simulink model "simulation_base"  (R2013a)
settings: Solver=ode4  StartTime=0.0  StopTime=10  FixedStep=Ts  RelTol=1e-3
values from neighbouring files (symbols this model uses):
  Cdc = 5e-3    (= 0.005)    [rpg_simulation_base.m]
  Crpcu_each = 1/(2*pi*fs*Zrpcu_each)    [rpg_simulation_base.m]
  ESR = 1e-3    (= 0.001)    [rpg_simulation_base.m]
  fs = 50    [rpg_loss_calculation.m]    (also in rpg_simulation_base.m)
  Lload = Xload/wout    [rpg_simulation_base.m]
  Ls = 1e-3    (= 0.001)    [rpg_simulation_base.m]
  Ppv = 40e3    (= 40000)    [rpg_simulation_base.m]
  Qpv = 30e3    (= 30000)    [rpg_simulation_base.m]
  Rload = Zload*pf    [rpg_simulation_base.m]
  RLs = 10e-3    (= 0.01)    [rpg_simulation_base.m]
  Rseries = 5    [rpg_simulation_base.m]
  Ts = 1e-5    (= 1e-05)    [rpg_simulation_base.m]
  V1 = Vdc*(Rseries+Rrefl)/Rrefl    (= 1083.33333333)    [rpg_simulation_base.m]
  Vdc = 750    [calculate_loss.m]    (also in rpg_loss_calculation.m; rpg_simulation_base.m)
  Vline = 400    [calculate_loss.m]    (also in rpg_loss_calculation.m; rpg_simulation_base.m = 34500)
  Vphase = 400/sqrt(3)    [rpg_simulation_base.m]
  Xs = 2*pi*fs*Ls    (= 0.314159265359)    [rpg_simulation_base.m]
undefined symbols (not defined in the file or in its folder): rpcu_s1, rpcu_s2, rpcu_s3, rpcu_s4
libraries: powerlib x74, powerlib_meascontrol x13, simulink x1
settings Model: Creator=hp  LastModifiedBy=ugurm

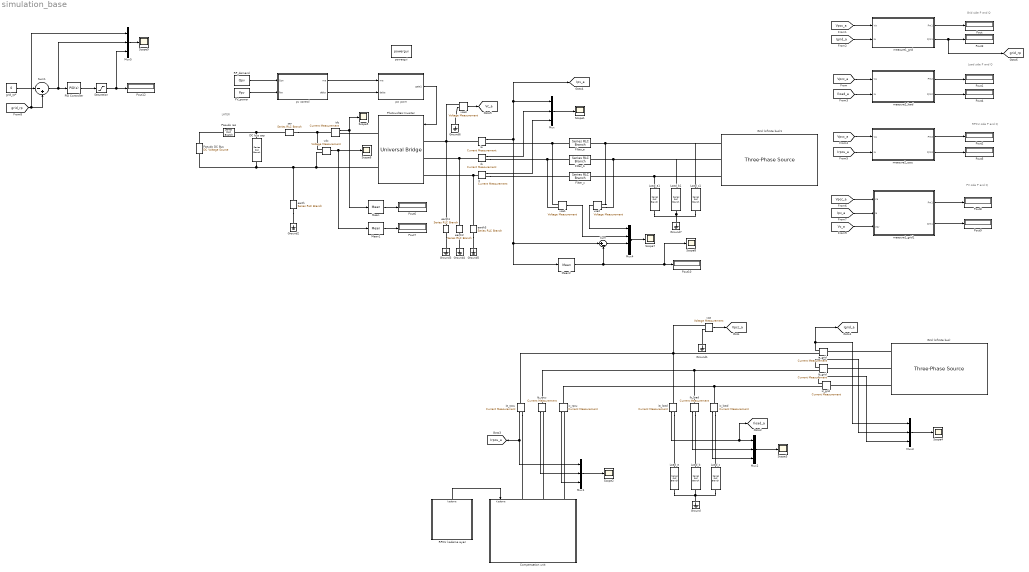
== system simulation_base ==
  note: LATER
  note: Grid side P and Q
  note: Load side P and Q
  note: RPCU side P and Q
  note: PV side P and Q
  Compensation unit : Subsystem
  DC bus cap : powerlib/Elements/Series RLC Branch  LConnTagsString=__new0  RConnTagsString=__new0  BranchType=RC  Resistance=ESR  Inductance=1e-3  SetiL0=off  InitialCurrent=0  Capacitance=Cdc  Setx0=on  InitialVoltage=600  Measurements=None
  Filter_a : powerlib/Elements/Series RLC Branch  LConnTagsString=__new0  RConnTagsString=__new0  BranchType=RL  Resistance=RLs  Inductance=Ls  SetiL0=off  InitialCurrent=0  Capacitance=1e-6  Setx0=off  InitialVoltage=0  Measurements=None
  Filter_b : powerlib/Elements/Series RLC Branch  LConnTagsString=__new0  RConnTagsString=__new0  BranchType=RL  Resistance=RLs  Inductance=Ls  SetiL0=off  InitialCurrent=0  Capacitance=1e-6  Setx0=off  InitialVoltage=0  Measurements=None
  Filter_c : powerlib/Elements/Series RLC Branch  LConnTagsString=__new0  RConnTagsString=__new0  BranchType=RL  Resistance=RLs  Inductance=Ls  SetiL0=off  InitialCurrent=0  Capacitance=1e-6  Setx0=off  InitialVoltage=0  Measurements=None
  Grid (infinite bus) : powerlib/Electrical Sources/Three-Phase Source  Voltage=Vline  PhaseAngle=0  Frequency=fs  InternalConnection=Yg  SpecifyImpedance=off  Resistance=0  Inductance=0  ShortCircuitLevel=100e6  BaseVoltage=Vline  XRratio=7  BusType=swing  Pref=0  Qref=0  Qmin=-inf  Qmax=inf
  Grid (infinite bus)1 : powerlib/Electrical Sources/Three-Phase Source  Voltage=Vline  PhaseAngle=0  Frequency=fs  InternalConnection=Yg  SpecifyImpedance=off  Resistance=1e-3  Inductance=1e-6  ShortCircuitLevel=100e6  BaseVoltage=Vline  XRratio=7  BusType=swing  Pref=0  Qref=0  Qmin=-inf  Qmax=inf
  Ground{,1..7} (8 alike) : powerlib/Elements/Ground  LConnTagsString=a
  Load_a : powerlib/Elements/Series RLC Branch  LConnTagsString=__new0  RConnTagsString=__new0  BranchType=RL  Resistance=Rload  Inductance=Lload  SetiL0=off  InitialCurrent=0  Capacitance=1e-6  Setx0=off  InitialVoltage=0  Measurements=None
  Load_a1 : powerlib/Elements/Series RLC Branch  LConnTagsString=__new0  RConnTagsString=__new0  BranchType=RL  Resistance=Rload  Inductance=Lload  SetiL0=off  InitialCurrent=0  Capacitance=1e-6  Setx0=off  InitialVoltage=0  Measurements=None
  Load_b : powerlib/Elements/Series RLC Branch  LConnTagsString=__new0  RConnTagsString=__new0  BranchType=RL  Resistance=Rload  Inductance=Lload  SetiL0=off  InitialCurrent=0  Capacitance=1e-6  Setx0=off  InitialVoltage=0  Measurements=None
  Load_b1 : powerlib/Elements/Series RLC Branch  LConnTagsString=__new0  RConnTagsString=__new0  BranchType=RL  Resistance=Rload  Inductance=Lload  SetiL0=off  InitialCurrent=0  Capacitance=1e-6  Setx0=off  InitialVoltage=0  Measurements=None
  Load_c : powerlib/Elements/Series RLC Branch  LConnTagsString=__new0  RConnTagsString=__new0  BranchType=RL  Resistance=Rload  Inductance=Lload  SetiL0=off  InitialCurrent=0  Capacitance=1e-6  Setx0=off  InitialVoltage=0  Measurements=None
  Load_c1 : powerlib/Elements/Series RLC Branch  LConnTagsString=__new0  RConnTagsString=__new0  BranchType=RL  Resistance=Rload  Inductance=Lload  SetiL0=off  InitialCurrent=0  Capacitance=1e-6  Setx0=off  InitialVoltage=0  Measurements=None
  Mean : powerlib_meascontrol/Measurements/Mean  Freq=1e3  Vinit=0  Ts=0
  Mean1 : powerlib_meascontrol/Measurements/Mean  Freq=1e3  Vinit=0  Ts=0
  Mean2 : powerlib_meascontrol/Measurements/Mean  Freq=50  Vinit=0  Ts=0
  Mux{,1..3,5} (5 alike) : Mux  Inputs=3
  Mux4 : Mux
  PID Controller : simulink/Continuous/PID Controller  Controller=PID  TimeDomain=Continuous-time  SampleTime=1  IntegratorMethod=Forward Euler  FilterMethod=Forward Euler  Form=Parallel  P=1  I=1  D=0  N=100  InitialConditionSource=internal  InitialConditionForIntegrator=0  InitialConditionForFilter=0  ExternalReset=none  LimitOutput=off  UpperSaturationLimit=inf  LowerSaturationLimit=-inf  LinearizeAsGain=on  AntiWindupMode=none  Kb=1  TrackingMode=off  Kt=1  PParamMin=[]  PParamMax=[]  IParamMin=[]  IParamMax=[]  DParamMin=[]  DParamMax=[]  NParamMin=[]  NParamMax=[]  KbParamMin=[]  KbParamMax=[]  KtParamMin=[]  KtParamMax=[]  POutMin=[]  POutMax=[]  IOutMin=[]  IOutMax=[]  DOutMin=[]  DOutMax=[]  NOutMin=[]  NOutMax=[]  KbOutMin=[]  KbOutMax=[]  KtOutMin=[]  KtOutMax=[]  IntegratorOutMin=[]  IntegratorOutMax=[]  FilterOutMin=[]  FilterOutMax=[]  SumOutMin=[]  SumOutMax=[]  SumI1OutMin=[]  SumI1OutMax=[]  SumI2OutMin=[]  SumI2OutMax=[]  SumI3OutMin=[]  SumI3OutMax=[]  SumDOutMin=[]  SumDOutMax=[]  SaturationOutMin=[]  SaturationOutMax=[]  IntegratorContinuousStateAttributes=''  IntegratorStateMustResolveToSignalObject=off  IntegratorRTWStateStorageClass=Auto  FilterContinuousStateAttributes=''  FilterStateMustResolveToSignalObject=off  FilterRTWStateStorageClass=Auto
  PV_power : Constant  Value=Ppv
  Photovoltaic Inverter : powerlib/Power Electronics/Universal Bridge  Arms=3  SnubberResistance=1e5  SnubberCapacitance=inf  Device=IGBT / Diodes  Ron=1e-3  Lon=0  ForwardVoltages="[  0  0  ]"  ForwardVoltage=0  GTOparameters=[ 10e-6 , 20e-6 ]  IGBTparameters=[ 1e-6 , 2e-6 ]  Measurements=None  Measurements_2=None  converterType=Rectifier
  Pout{,1..10,12} (12 alike) : Display
      Pout settings: Format=bank
      Pout1 settings: Format=bank
      Pout10 settings: Format=bank
      Pout2 settings: Format=bank
      Pout3 settings: Format=bank
      Pout4 settings: Format=bank
      Pout5 settings: Format=bank
      Pout6 settings: Format=bank
      Pout7 settings: Format=bank
      Pout8 settings: Format=bank
      Pout9 settings: Format=bank
  Pseudo DC Bus : powerlib/Electrical Sources/DC Voltage Source  Amplitude=V1  Measurements=None
  Pseudo res : powerlib/Elements/Series RLC Branch  LConnTagsString=__new0  RConnTagsString=__new0  BranchType=R  Resistance=Rseries  Inductance=1e-3  SetiL0=off  InitialCurrent=0  Capacitance=3e-3  Setx0=off  InitialVoltage=0  Measurements=None
  RPCU kademe ayari : Subsystem
  RP_demand : Constant  Value=Qpv
  Saturation : Saturate  UpperLimit=100000  LowerLimit=0
  Scope{1..9} (9 alike) : Scope
      Scope1 settings: YMin=-300  YMax=300
      Scope2 settings: YMin=-110  YMax=110  SaveName=ScopeData2
      Scope3 settings: YMin=-500  YMax=500  SaveName=ScopeData3
      Scope4 settings: YMin=-500  YMax=500  SaveName=ScopeData5
      Scope5 settings: YMin=-40  YMax=110
      Scope6 settings: YMin=602  YMax=619  SaveName=ScopeData7
      Scope7 settings: YMin=-800  YMax=800  SaveName=ScopeData6
      Scope8 settings: YMin=-77  YMax=-57  SaveName=ScopeData8
      Scope9 settings: YMin=74000  YMax=89000  SaveName=ScopeData9
  Sum : Sum  Inputs=|+-
  Sum1 : Sum  Inputs=|-+
  earth{,1..3} (4 alike) : powerlib/Elements/Series RLC Branch  LConnTagsString=__new0  RConnTagsString=__new0  BranchType=R  Resistance=1e12  Inductance=Lload  SetiL0=off  InitialCurrent=0  Capacitance=1e-6  Setx0=off  InitialVoltage=0  Measurements=None
  grid_rp* : Constant  Value=0
  ia : powerlib/Measurements/Current Measurement  PhasorSimulation=off  OutputType=Complex  PSBequivalent=0
  ia_grid : powerlib/Measurements/Current Measurement  PhasorSimulation=off  OutputType=Complex  PSBequivalent=0
  ia_load : powerlib/Measurements/Current Measurement  PhasorSimulation=off  OutputType=Complex  PSBequivalent=0
  ia_rpcu : powerlib/Measurements/Current Measurement  PhasorSimulation=off  OutputType=Complex  PSBequivalent=0
  ib : powerlib/Measurements/Current Measurement  PhasorSimulation=off  OutputType=Complex  PSBequivalent=0
  ib_grid : powerlib/Measurements/Current Measurement  PhasorSimulation=off  OutputType=Complex  PSBequivalent=0
  ib_load : powerlib/Measurements/Current Measurement  PhasorSimulation=off  OutputType=Complex  PSBequivalent=0
  ib_rpcu : powerlib/Measurements/Current Measurement  PhasorSimulation=off  OutputType=Complex  PSBequivalent=0
  ic : powerlib/Measurements/Current Measurement  PhasorSimulation=off  OutputType=Complex  PSBequivalent=0
  ic_grid : powerlib/Measurements/Current Measurement  PhasorSimulation=off  OutputType=Complex  PSBequivalent=0
  ic_load : powerlib/Measurements/Current Measurement  PhasorSimulation=off  OutputType=Complex  PSBequivalent=0
  ic_rpcu : powerlib/Measurements/Current Measurement  PhasorSimulation=off  OutputType=Complex  PSBequivalent=0
  idc : powerlib/Measurements/Current Measurement  PhasorSimulation=off  OutputType=Complex  PSBequivalent=0
  measure1_grid : Subsystem
  measure1_grid1 : Subsystem
  measure2_load : Subsystem
  measure2_rpcu : Subsystem
  powergui : powerlib/powergui  Priority=1  SimulationMode=Discrete  SolverType=Tustin  SampleTime=Ts  frequency=60  SPID=off  DisableSnubberDevices=off  DisableRonSwitches=off  DisableVfSwitches=off  SwTol=0  Interpol=off  DisplayEquations=off  frequencyindice=0  Pbase=100e6  ErrMax=1e-4  Iterations=50  UnitsV=kV  UnitsW=MW  FunctionMessages=off  echomessages=off  HookPort=off  EnableUseOfTLC=off  x0status=blocks  RestoreLinks=warning  ResistiveCurrentMeasurement=off  Frange=[0:2:500]  Ylog=off  Xlog=on  ShowGrid=off  save=off  variable=ZData  ZoomFFT=off  StartTime=0.0  cycles=1  DisplayStyle=1  fundamental=60  FreqAxis=off  MaxFrequency=1000  frequencyindicesteady=1  RmsSteady=1  display=off  Ts=0  methode=off
  pv control : Subsystem
  pw pwm : Subsystem
  ser : powerlib/Elements/Series RLC Branch  LConnTagsString=__new0  RConnTagsString=__new0  BranchType=R  Resistance=1e-6  Inductance=Lload  SetiL0=off  InitialCurrent=0  Capacitance=1e-6  Setx0=off  InitialVoltage=0  Measurements=None
  vdc : powerlib/Measurements/Voltage Measurement  PhasorSimulation=off  OutputType=Complex  PSBequivalent=0
  vsa{,1..3} (4 alike) : powerlib/Measurements/Voltage Measurement  PhasorSimulation=off  OutputType=Complex  PSBequivalent=0
  tag scope: Igrid_a=global, Iload_a=global, Ipv_a=global, Irpcu_a=global, Vc_a=global, Vpcc_a=global, grid_rp=global
  wires:
  RPCU kademe ayari/1(kademe) -> Compensation unit/1(Kademe)
  ia/1 -> Sum/1, Mean2/1, [Ipv_a], Mux/1
  ib/1 -> Mux/2
  ic/1 -> Mux/3
  Mux/1 -> Scope1/1
  pw pwm/1(gate1) -> Photovoltaic Inverter/1
  Mux1/1 -> Scope2/1
  ib_rpcu/1 -> Mux1/2
  ic_rpcu/1 -> Mux1/3
  Mux2/1 -> Scope3/1
  ia_load/1 -> [Iload_a], Mux2/1
  ib_load/1 -> Mux2/2
  ic_load/1 -> Mux2/3
  Mux3/1 -> Scope4/1
  ib_grid/1 -> Mux3/2
  ic_grid/1 -> Mux3/3
  ia_grid/1 -> [Igrid_a], Mux3/1
  vdc/1 -> Mean1/1, Scope6/1
  vsa/1 -> [Vpcc_a]
  [Vpcc_a] -> measure2_load/1(Va)
  [Vpcc_a] -> measure1_grid/1(Va)
  [Igrid_a] -> measure1_grid/2(Ia)
  [Iload_a] -> measure2_load/2(Ia)
  [Vpcc_a] -> measure2_rpcu/1(Va)
  [Irpcu_a] -> measure2_rpcu/2(Ia)
  ia_rpcu/1 -> [Irpcu_a], Mux1/1
  measure1_grid/1(Pm1) -> Pout/1
  measure2_load/1(Pm2) -> Pout1/1
  measure2_rpcu/1(Pm3) -> Pout2/1
  measure1_grid/2(Qm1) -> [grid_rp], Pout3/1
  measure2_load/2(Qm2) -> Pout4/1
  measure2_rpcu/2(Qm3) -> Pout5/1
  idc/1 -> Scope5/1, Mean/1
  Mean/1 -> Pout6/1
  Mean1/1 -> Pout7/1
  Mux4/1 -> Scope7/1
  vsa2/1 -> Mux4/1
  vsa1/1 -> Mux4/2
  Sum/1 -> Mux4/3
  ? -> Mux4/4
  Mean2/1 -> Sum/2, Scope8/1, Pout10/1
  vsa3/1 -> [Vc_a]
  [Vpcc_a] -> measure1_grid1/1(Va)
  [Ipv_a] -> measure1_grid1/2(Ia)
  measure1_grid1/1(Pm1) -> Pout8/1
  measure1_grid1/2(Qm1) -> Pout9/1
  [Vc_a] -> measure1_grid1/3(Vpv)
  grid_rp*/1 -> Sum1/1
  [grid_rp] -> Sum1/2, Mux5/1
  Sum1/1 -> Mux5/2, PID Controller/1
  PID Controller/1 -> Saturation/1
  PV_power/1 -> pv control/2(Ppv)
  Saturation/1 -> Pout12/1, Mux5/3
  Mux5/1 -> Scope9/1
  pv control/1(ma) -> pw pwm/1(ma)
  pv control/2(delta) -> pw pwm/2(delta)
  RP_demand/1 -> pv control/1(Qpv)
  connections:
  Photovoltaic Inverter/RConn2 -- DC bus cap/RConn1 -- Pseudo DC Bus/LConn1 -- earth/LConn1 -- vdc/LConn2
  Pseudo res/RConn1 -- Pseudo DC Bus/RConn1
  DC bus cap/LConn1 -- ser/RConn1 -- Pseudo res/LConn1
  ia/LConn1 -- vsa3/LConn1 -- Photovoltaic Inverter/LConn1 -- earth1/LConn1
  Filter_a/LConn1 -- ia/RConn1 -- vsa1/LConn1
  ib/LConn1 -- earth2/LConn1 -- Photovoltaic Inverter/LConn2
  ib/RConn1 -- vsa1/LConn2 -- Filter_b/LConn1
  ic/LConn1 -- Photovoltaic Inverter/LConn3 -- earth3/LConn1
  ic/RConn1 -- Filter_c/LConn1
  ia_load/RConn1 -- Load_a/LConn1
  ic_load/RConn1 -- Load_c/LConn1
  ib_load/RConn1 -- Load_b/LConn1
  Ground/LConn1 -- Load_a/RConn1 -- Load_c/RConn1 -- Load_b/RConn1
  Ground1/LConn1 -- vsa/LConn2
  ic_load/LConn1 -- ic_grid/RConn1 -- ic_rpcu/LConn1
  ib_load/LConn1 -- ib_rpcu/LConn1 -- ib_grid/RConn1
  ia_load/LConn1 -- ia_rpcu/LConn1 -- vsa/LConn1 -- ia_grid/RConn1
  Grid (infinite bus)/RConn1 -- ia_grid/LConn1
  Grid (infinite bus)/RConn2 -- ib_grid/LConn1
  Grid (infinite bus)/RConn3 -- ic_grid/LConn1
  Compensation unit/LConn2 -- ib_rpcu/RConn1
  Compensation unit/LConn3 -- ic_rpcu/RConn1
  ia_rpcu/RConn1 -- Compensation unit/LConn1
  vsa2/LConn1 -- Grid (infinite bus)1/RConn1 -- Load_c1/LConn1 -- Filter_a/RConn1
  vsa2/LConn2 -- Grid (infinite bus)1/RConn2 -- Load_b1/LConn1 -- Filter_b/RConn1
  Load_a1/LConn1 -- Filter_c/RConn1 -- Grid (infinite bus)1/RConn3
  vdc/LConn1 -- ser/LConn1 -- idc/LConn1
  Photovoltaic Inverter/RConn1 -- idc/RConn1
  earth/RConn1 -- Ground2/LConn1
  earth1/RConn1 -- Ground3/LConn1
  earth2/RConn1 -- Ground4/LConn1
  earth3/RConn1 -- Ground5/LConn1
  Ground6/LConn1 -- vsa3/LConn2
  Load_b1/RConn1 -- Load_a1/RConn1 -- Ground7/LConn1 -- Load_c1/RConn1

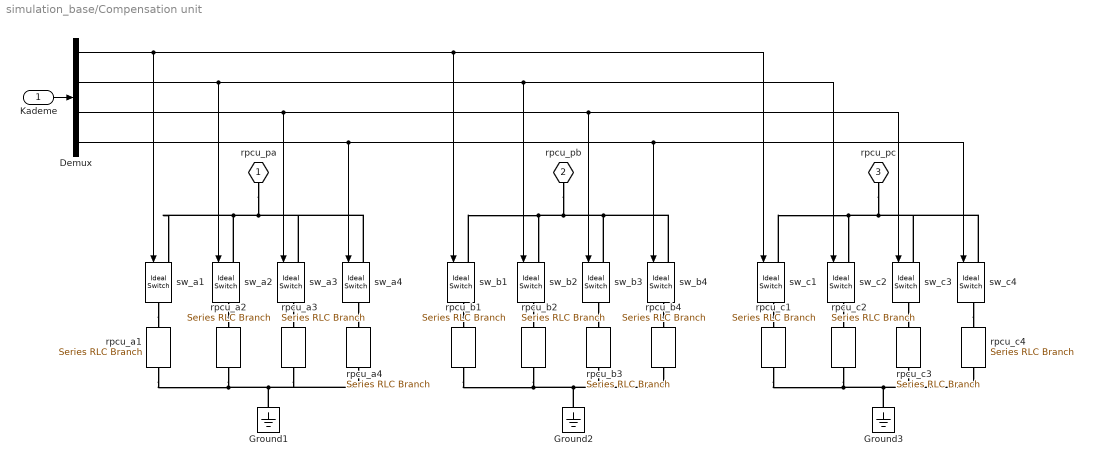
== system simulation_base/Compensation unit ==
  Kademe : Inport
  " sw_a2" : powerlib/Power Electronics/Ideal Switch  Ron=0.001  Lon=0  IC=0  Rs=inf  Cs=inf  Measurements=off
  Demux : Demux
  Ground1 : powerlib/Elements/Ground  LConnTagsString=a
  Ground2 : powerlib/Elements/Ground  LConnTagsString=a
  Ground3 : powerlib/Elements/Ground  LConnTagsString=a
  rpcu_a{1..4} (4 alike) : powerlib/Elements/Series RLC Branch  LConnTagsString=__new0  RConnTagsString=__new0  BranchType=C  Resistance=1e9  Inductance=1e-6  SetiL0=off  InitialCurrent=0  Capacitance=Crpcu_each  Setx0=off  InitialVoltage=0  Measurements=None
  rpcu_b{1..4} (4 alike) : powerlib/Elements/Series RLC Branch  LConnTagsString=__new0  RConnTagsString=__new0  BranchType=C  Resistance=1e9  Inductance=1e-6  SetiL0=off  InitialCurrent=0  Capacitance=Crpcu_each  Setx0=off  InitialVoltage=0  Measurements=None
  rpcu_c{1..4} (4 alike) : powerlib/Elements/Series RLC Branch  LConnTagsString=__new0  RConnTagsString=__new0  BranchType=C  Resistance=1e9  Inductance=1e-6  SetiL0=off  InitialCurrent=0  Capacitance=Crpcu_each  Setx0=off  InitialVoltage=0  Measurements=None
  sw_a1 : powerlib/Power Electronics/Ideal Switch  Ron=0.001  Lon=0  IC=0  Rs=inf  Cs=inf  Measurements=off
  sw_a3 : powerlib/Power Electronics/Ideal Switch  Ron=0.001  Lon=0  IC=0  Rs=inf  Cs=inf  Measurements=off
  sw_a4 : powerlib/Power Electronics/Ideal Switch  Ron=0.001  Lon=0  IC=0  Rs=inf  Cs=inf  Measurements=off
  sw_b{1..4} (4 alike) : powerlib/Power Electronics/Ideal Switch  Ron=0.001  Lon=0  IC=0  Rs=inf  Cs=inf  Measurements=off
  sw_c{1..4} (4 alike) : powerlib/Power Electronics/Ideal Switch  Ron=0.001  Lon=0  IC=0  Rs=inf  Cs=inf  Measurements=off
  rpcu_pa : PMIOPort  Port=1  Side=Left
  rpcu_pb : PMIOPort  Port=2  Side=Left
  rpcu_pc : PMIOPort  Port=3  Side=Left
  wires:
  Kademe/1 -> Demux/1
  Demux/1 -> sw_c1/1, sw_b1/1, sw_a1/1
  Demux/2 -> sw_b2/1, sw_c2/1, " sw_a2"/1
  Demux/3 -> sw_c3/1, sw_b3/1, sw_a3/1
  Demux/4 -> sw_c4/1, sw_b4/1, sw_a4/1
  connections:
  Ground1/LConn1 -- rpcu_a2/RConn1 -- rpcu_a1/RConn1 -- rpcu_a4/RConn1 -- rpcu_a3/RConn1
  " sw_a2"/LConn1 -- rpcu_pa/RConn1 -- sw_a3/LConn1 -- sw_a4/LConn1 -- sw_a1/LConn1
  sw_a3/RConn1 -- rpcu_a3/LConn1
  " sw_a2"/RConn1 -- rpcu_a2/LConn1
  sw_a4/RConn1 -- rpcu_a4/LConn1
  rpcu_b1/RConn1 -- rpcu_b4/RConn1 -- rpcu_b3/RConn1 -- Ground2/LConn1 -- rpcu_b2/RConn1
  sw_b4/LConn1 -- sw_b3/LConn1 -- rpcu_pb/RConn1 -- sw_b2/LConn1 -- sw_b1/LConn1
  sw_b1/RConn1 -- rpcu_b1/LConn1
  sw_b4/RConn1 -- rpcu_b4/LConn1
  sw_b3/RConn1 -- rpcu_b3/LConn1
  sw_b2/RConn1 -- rpcu_b2/LConn1
  sw_c3/RConn1 -- rpcu_c3/LConn1
  sw_c1/RConn1 -- rpcu_c1/LConn1
  sw_c4/RConn1 -- rpcu_c4/LConn1
  sw_c2/RConn1 -- rpcu_c2/LConn1
  sw_c1/LConn1 -- rpcu_pc/RConn1 -- sw_c3/LConn1 -- sw_c4/LConn1 -- sw_c2/LConn1
  rpcu_c1/RConn1 -- rpcu_c2/RConn1 -- Ground3/LConn1 -- rpcu_c4/RConn1 -- rpcu_c3/RConn1
  sw_a1/RConn1 -- rpcu_a1/LConn1

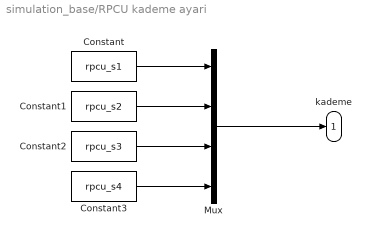
== system simulation_base/RPCU kademe ayari ==
  Constant : Constant  Value=rpcu_s1
  Constant1 : Constant  Value=rpcu_s2
  Constant2 : Constant  Value=rpcu_s3
  Constant3 : Constant  Value=rpcu_s4
  Mux : Mux
  kademe : Outport
  wires:
  Constant1/1 -> Mux/2
  Constant/1 -> Mux/1
  Mux/1 -> kademe/1
  Constant3/1 -> Mux/4
  Constant2/1 -> Mux/3

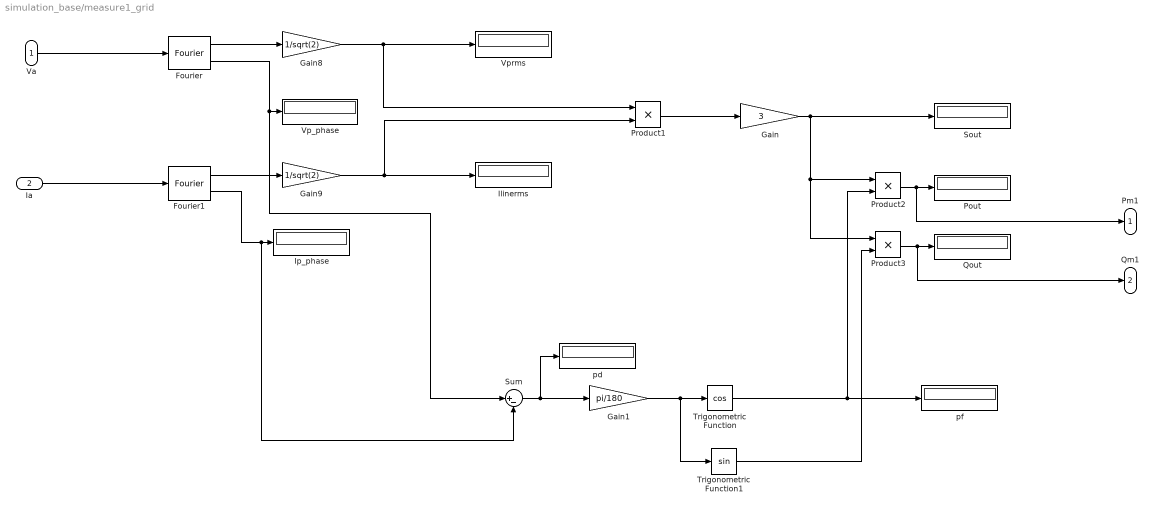
== system simulation_base/measure1_grid ==
  Va : Inport
  Ia : Inport  Port=2
  Fourier : powerlib_meascontrol/Measurements/Fourier  Freq=50  n=1  InInit=[0, 0]  Ts=0
  Fourier1 : powerlib_meascontrol/Measurements/Fourier  Freq=50  n=1  InInit=[0, 0]  Ts=0
  Gain : Gain  Gain=3
  Gain1 : Gain  Gain=pi/180
  Gain8 : Gain  Gain=1/sqrt(2)
  Gain9 : Gain  Gain=1/sqrt(2)
  "Ilinerms " : Display
  Ip_phase : Display
  Pout : Display
  Product1 : Product
  Product2 : Product
  Product3 : Product
  Qout : Display
  Sout : Display
      settings: Format=short_e
  Sum : Sum  Inputs=|+-
  Trigonometric Function : Trigonometry  Operator=cos
  Trigonometric Function1 : Trigonometry
  Vp_phase : Display
  "Vprms " : Display
  pd : Display
  pf : Display
  Pm1 : Outport
  Qm1 : Outport  Port=2
  wires:
  Gain8/1 -> "Vprms "/1, Product1/1
  Ia/1 -> Fourier1/1
  Fourier1/1 -> Gain9/1
  Va/1 -> Fourier/1
  Fourier/1 -> Gain8/1
  Product1/1 -> Gain/1
  Gain/1 -> Sout/1, Product2/1, Product3/1
  Trigonometric Function/1 -> pf/1, Product2/2
  Gain1/1 -> Trigonometric Function1/1, Trigonometric Function/1
  Product2/1 -> Pm1/1, Pout/1
  Fourier/2 -> Sum/1, Vp_phase/1
  Gain9/1 -> "Ilinerms "/1, Product1/2
  Fourier1/2 -> Sum/2, Ip_phase/1
  Sum/1 -> Gain1/1, pd/1
  Trigonometric Function1/1 -> Product3/2
  Product3/1 -> Qm1/1, Qout/1

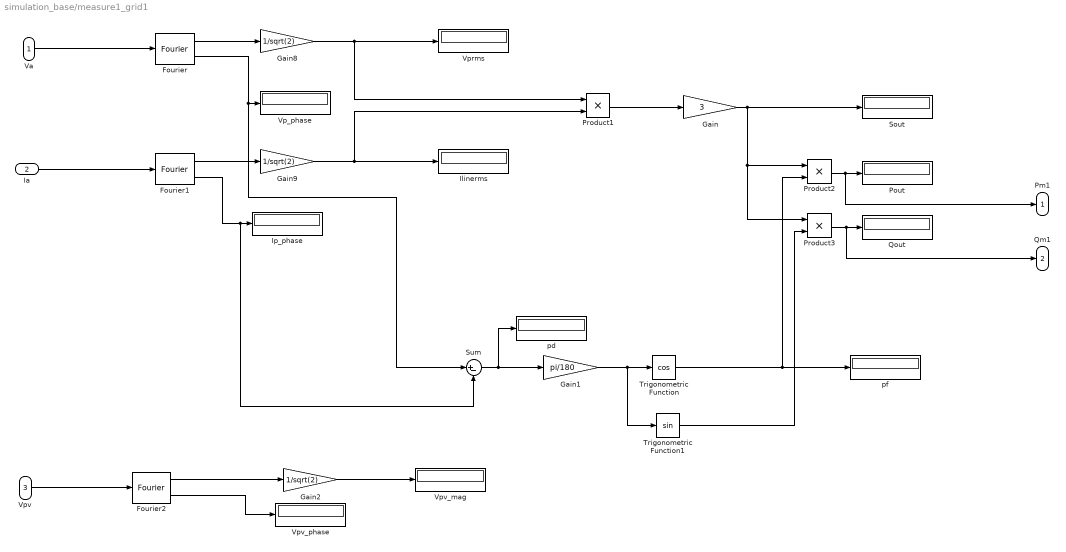
== system simulation_base/measure1_grid1 ==
  Va : Inport
  Ia : Inport  Port=2
  Vpv : Inport  Port=3
  Fourier : powerlib_meascontrol/Measurements/Fourier  Freq=50  n=1  InInit=[0, 0]  Ts=0
  Fourier1 : powerlib_meascontrol/Measurements/Fourier  Freq=50  n=1  InInit=[0, 0]  Ts=0
  Fourier2 : powerlib_meascontrol/Measurements/Fourier  Freq=50  n=1  InInit=[0, 0]  Ts=0
  Gain : Gain  Gain=3
  Gain1 : Gain  Gain=pi/180
  Gain2 : Gain  Gain=1/sqrt(2)
  Gain8 : Gain  Gain=1/sqrt(2)
  Gain9 : Gain  Gain=1/sqrt(2)
  "Ilinerms " : Display
  Ip_phase : Display
  Pout : Display
  Product1 : Product
  Product2 : Product
  Product3 : Product
  Qout : Display
  Sout : Display
      settings: Format=short_e
  Sum : Sum  Inputs=|+-
  Trigonometric Function : Trigonometry  Operator=cos
  Trigonometric Function1 : Trigonometry
  Vp_phase : Display
  "Vprms " : Display
  Vpv_mag : Display
  Vpv_phase : Display
  pd : Display
  pf : Display
  Pm1 : Outport
  Qm1 : Outport  Port=2
  wires:
  Gain8/1 -> "Vprms "/1, Product1/1
  Ia/1 -> Fourier1/1
  Fourier1/1 -> Gain9/1
  Va/1 -> Fourier/1
  Fourier/1 -> Gain8/1
  Product1/1 -> Gain/1
  Gain/1 -> Sout/1, Product2/1, Product3/1
  Trigonometric Function/1 -> pf/1, Product2/2
  Gain1/1 -> Trigonometric Function1/1, Trigonometric Function/1
  Product2/1 -> Pm1/1, Pout/1
  Fourier/2 -> Sum/1, Vp_phase/1
  Gain9/1 -> "Ilinerms "/1, Product1/2
  Fourier1/2 -> Sum/2, Ip_phase/1
  Sum/1 -> Gain1/1, pd/1
  Trigonometric Function1/1 -> Product3/2
  Product3/1 -> Qm1/1, Qout/1
  Fourier2/1 -> Gain2/1
  Fourier2/2 -> Vpv_phase/1
  Gain2/1 -> Vpv_mag/1
  Vpv/1 -> Fourier2/1

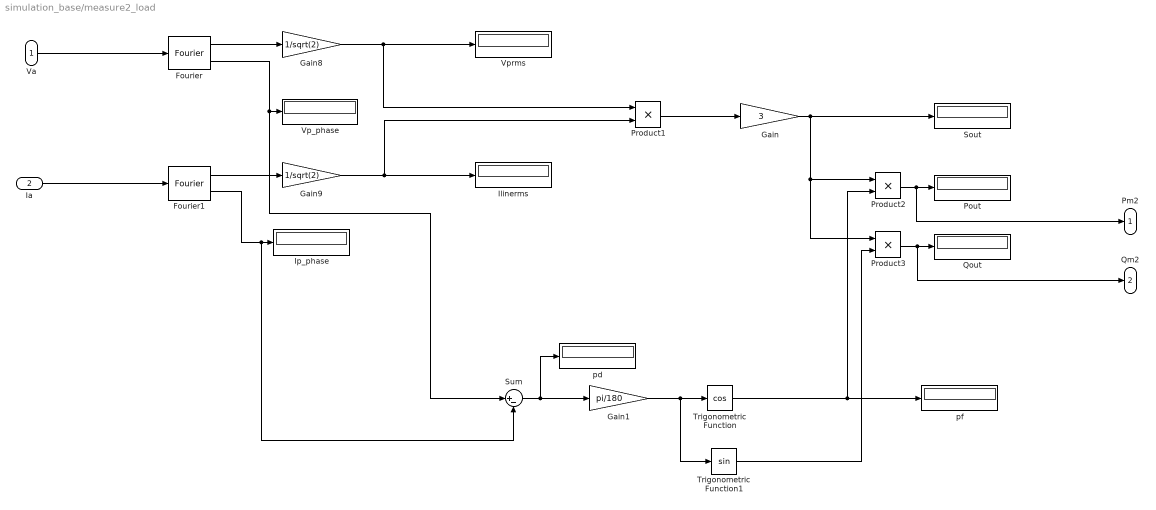
== system simulation_base/measure2_load ==
  Va : Inport
  Ia : Inport  Port=2
  Fourier : powerlib_meascontrol/Measurements/Fourier  Freq=50  n=1  InInit=[0, 0]  Ts=0
  Fourier1 : powerlib_meascontrol/Measurements/Fourier  Freq=50  n=1  InInit=[0, 0]  Ts=0
  Gain : Gain  Gain=3
  Gain1 : Gain  Gain=pi/180
  Gain8 : Gain  Gain=1/sqrt(2)
  Gain9 : Gain  Gain=1/sqrt(2)
  "Ilinerms " : Display
  Ip_phase : Display
  Pout : Display
  Product1 : Product
  Product2 : Product
  Product3 : Product
  Qout : Display
  Sout : Display
      settings: Format=short_e
  Sum : Sum  Inputs=|+-
  Trigonometric Function : Trigonometry  Operator=cos
  Trigonometric Function1 : Trigonometry
  Vp_phase : Display
  "Vprms " : Display
  pd : Display
  pf : Display
  Pm2 : Outport
  Qm2 : Outport  Port=2
  wires:
  Gain8/1 -> "Vprms "/1, Product1/1
  Ia/1 -> Fourier1/1
  Fourier1/1 -> Gain9/1
  Va/1 -> Fourier/1
  Fourier/1 -> Gain8/1
  Product1/1 -> Gain/1
  Gain/1 -> Sout/1, Product2/1, Product3/1
  Trigonometric Function/1 -> pf/1, Product2/2
  Gain1/1 -> Trigonometric Function1/1, Trigonometric Function/1
  Product2/1 -> Pm2/1, Pout/1
  Fourier/2 -> Sum/1, Vp_phase/1
  Gain9/1 -> "Ilinerms "/1, Product1/2
  Fourier1/2 -> Sum/2, Ip_phase/1
  Sum/1 -> Gain1/1, pd/1
  Trigonometric Function1/1 -> Product3/2
  Product3/1 -> Qm2/1, Qout/1

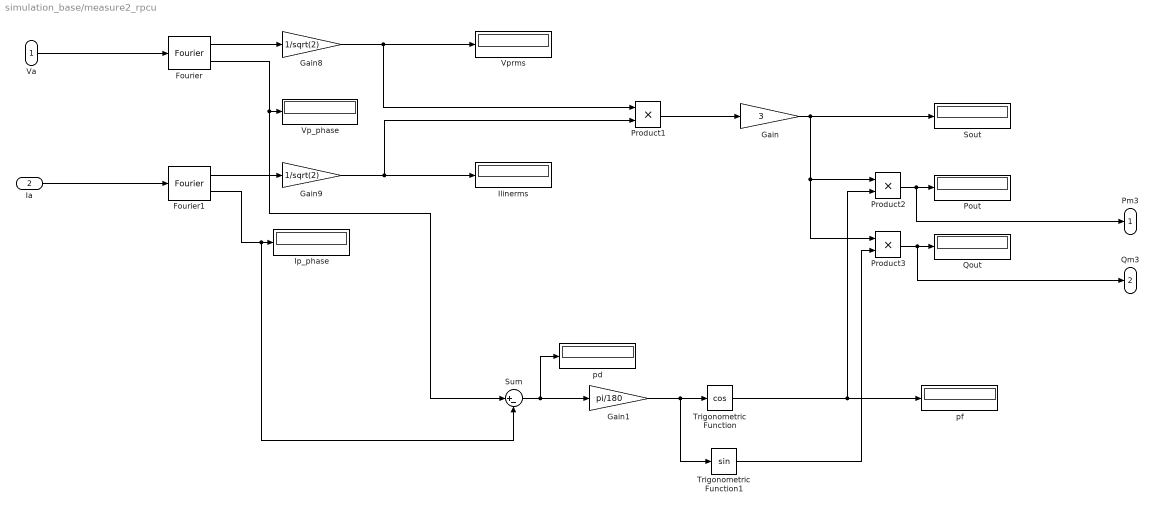
== system simulation_base/measure2_rpcu ==
  Va : Inport
  Ia : Inport  Port=2
  Fourier : powerlib_meascontrol/Measurements/Fourier  Freq=50  n=1  InInit=[0, 0]  Ts=0
  Fourier1 : powerlib_meascontrol/Measurements/Fourier  Freq=50  n=1  InInit=[0, 0]  Ts=0
  Gain : Gain  Gain=3
  Gain1 : Gain  Gain=pi/180
  Gain8 : Gain  Gain=1/sqrt(2)
  Gain9 : Gain  Gain=1/sqrt(2)
  "Ilinerms " : Display
  Ip_phase : Display
  Pout : Display
  Product1 : Product
  Product2 : Product
  Product3 : Product
  Qout : Display
  Sout : Display
      settings: Format=short_e
  Sum : Sum  Inputs=|+-
  Trigonometric Function : Trigonometry  Operator=cos
  Trigonometric Function1 : Trigonometry
  Vp_phase : Display
  "Vprms " : Display
  pd : Display
  pf : Display
  Pm3 : Outport
  Qm3 : Outport  Port=2
  wires:
  Gain8/1 -> "Vprms "/1, Product1/1
  Ia/1 -> Fourier1/1
  Fourier1/1 -> Gain9/1
  Va/1 -> Fourier/1
  Fourier/1 -> Gain8/1
  Product1/1 -> Gain/1
  Gain/1 -> Sout/1, Product2/1, Product3/1
  Trigonometric Function/1 -> pf/1, Product2/2
  Gain1/1 -> Trigonometric Function1/1, Trigonometric Function/1
  Product2/1 -> Pm3/1, Pout/1
  Fourier/2 -> Sum/1, Vp_phase/1
  Gain9/1 -> "Ilinerms "/1, Product1/2
  Fourier1/2 -> Sum/2, Ip_phase/1
  Sum/1 -> Gain1/1, pd/1
  Trigonometric Function1/1 -> Product3/2
  Product3/1 -> Qm3/1, Qout/1

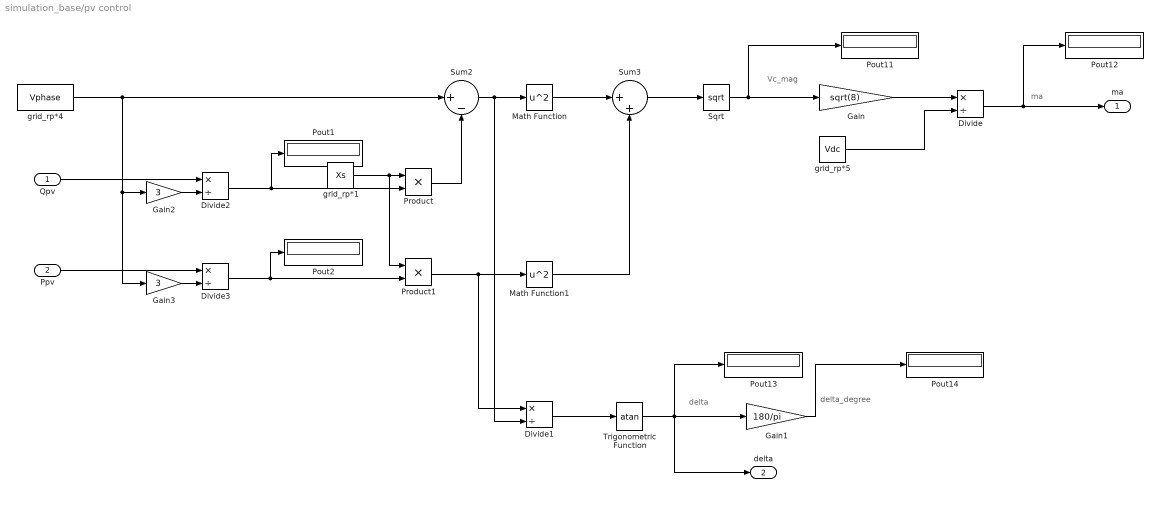
== system simulation_base/pv control ==
  note: delta_degree
  note: delta
  note: ma
  note: Vc_mag
  Qpv : Inport
  Ppv : Inport  Port=2
  Divide{,1..3} (4 alike) : Product  Inputs=*/
  Gain : Gain  Gain=sqrt(8)
  Gain1 : Gain  Gain=180/pi
  Gain2 : Gain  Gain=3
  Gain3 : Gain  Gain=3
  Math Function : Math  Operator=square  SaturateOnIntegerOverflow=on
  Math Function1 : Math  Operator=square  SaturateOnIntegerOverflow=on
  Pout{1..2,11..14} (6 alike) : Display
      Pout11 settings: Format=bank
  Product : Product
  Product1 : Product
  Sqrt : Sqrt  SaturateOnIntegerOverflow=on
  Sum2 : Sum  Inputs=|+-
  Sum3 : Sum  Inputs=|++
  Trigonometric Function : Trigonometry  Operator=atan  OutputSignalType=real
  grid_rp*1 : Constant  Value=Xs
  grid_rp*4 : Constant  Value=Vphase
  grid_rp*5 : Constant  Value=Vdc
  ma : Outport
  delta : Outport  Port=2
  wires:
  Product1/1 -> Divide1/1, Math Function1/1
  Divide2/1 -> Pout1/1, Product/2
  Gain/1 -> Divide/1
  Divide3/1 -> Pout2/1, Product1/2
  Product/1 -> Sum2/2
  Gain1/1 -> Pout14/1
  Sqrt/1 -> Gain/1, Pout11/1
  Math Function/1 -> Sum3/1
  Math Function1/1 -> Sum3/2
  Sum3/1 -> Sqrt/1
  Sum2/1 -> Divide1/2, Math Function/1
  grid_rp*5/1 -> Divide/2
  Trigonometric Function/1 -> delta/1, Pout13/1, Gain1/1
  Divide/1 -> ma/1, Pout12/1
  Divide1/1 -> Trigonometric Function/1
  grid_rp*1/1 -> Product1/1, Product/1
  Qpv/1 -> Divide2/1
  Gain2/1 -> Divide2/2
  grid_rp*4/1 -> Gain3/1, Gain2/1, Sum2/1
  Ppv/1 -> Divide3/1
  Gain3/1 -> Divide3/2

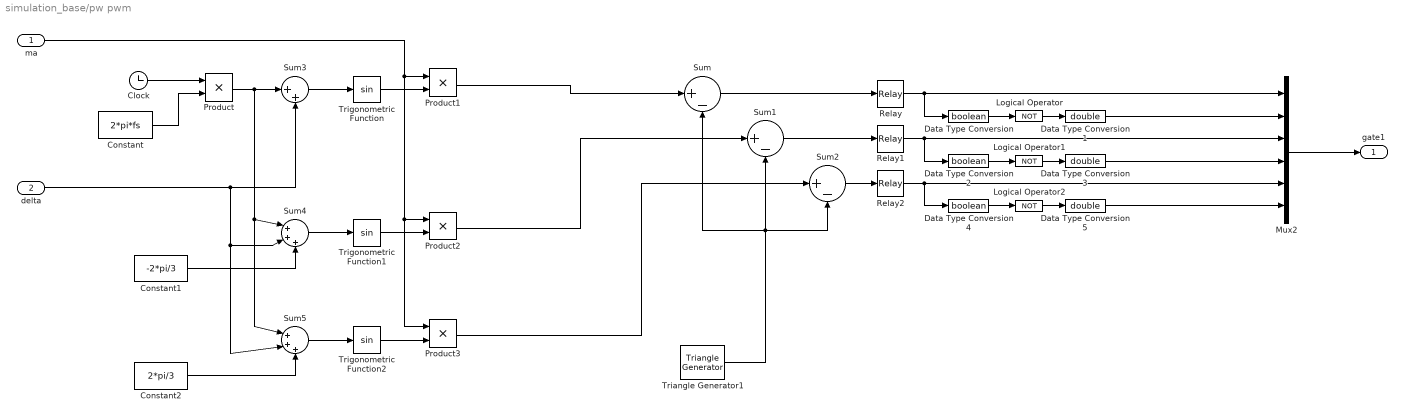
== system simulation_base/pw pwm ==
  ma : Inport
  delta : Inport  Port=2
  Clock : Clock
  Constant : Constant  Value=2*pi*fs
  Constant1 : Constant  Value=-2*pi/3
  Constant2 : Constant  Value=2*pi/3
  Data Type Conversion : DataTypeConversion  OutDataTypeStr=boolean
  Data Type Conversion1 : DataTypeConversion  OutDataTypeStr=double
  Data Type Conversion2 : DataTypeConversion  OutDataTypeStr=boolean
  Data Type Conversion3 : DataTypeConversion  OutDataTypeStr=double
  Data Type Conversion4 : DataTypeConversion  OutDataTypeStr=boolean
  Data Type Conversion5 : DataTypeConversion  OutDataTypeStr=double
  Logical Operator : Logic  Operator=NOT  AllPortsSameDT=off  OutDataTypeStr=boolean
  Logical Operator1 : Logic  Operator=NOT  AllPortsSameDT=off  OutDataTypeStr=boolean
  Logical Operator2 : Logic  Operator=NOT  AllPortsSameDT=off  OutDataTypeStr=boolean
  Mux2 : Mux  Inputs=6
  Product{,1..3} (4 alike) : Product
  Relay : Relay
  Relay1 : Relay
  Relay2 : Relay
  Sum : Sum  Inputs=|+-
  Sum1 : Sum  Inputs=|+-
  Sum2 : Sum  Inputs=|+-
  Sum3 : Sum  Inputs=|++
  Sum4 : Sum  Inputs=|+++
  Sum5 : Sum  Inputs=|+++
  Triangle Generator1 : powerlib_meascontrol/Pulse & Signal Generators/Triangle Generator  Freq=fsw  Phase=0  Ts=0
  Trigonometric Function : Trigonometry
  Trigonometric Function1 : Trigonometry
  Trigonometric Function2 : Trigonometry
  gate1 : Outport
  wires:
  Product1/1 -> Sum/1
  Triangle Generator1/1 -> Sum/2, Sum1/2, Sum2/2
  Product2/1 -> Sum1/1
  Product3/1 -> Sum2/1
  Sum/1 -> Relay/1
  Sum1/1 -> Relay1/1
  Sum2/1 -> Relay2/1
  Data Type Conversion/1 -> Logical Operator/1
  Relay/1 -> Data Type Conversion/1, Mux2/1
  Logical Operator/1 -> Data Type Conversion1/1
  Data Type Conversion1/1 -> Mux2/2
  Data Type Conversion2/1 -> Logical Operator1/1
  Relay1/1 -> Data Type Conversion2/1, Mux2/3
  Logical Operator1/1 -> Data Type Conversion3/1
  Data Type Conversion3/1 -> Mux2/4
  Data Type Conversion4/1 -> Logical Operator2/1
  Relay2/1 -> Data Type Conversion4/1, Mux2/5
  Logical Operator2/1 -> Data Type Conversion5/1
  Mux2/1 -> gate1/1
  Data Type Conversion5/1 -> Mux2/6
  Clock/1 -> Product/1
  Constant/1 -> Product/2
  Sum3/1 -> Trigonometric Function/1
  Trigonometric Function/1 -> Product1/2
  Constant1/1 -> Sum4/3
  Sum4/1 -> Trigonometric Function1/1
  Trigonometric Function1/1 -> Product2/2
  Product/1 -> Sum5/1, Sum4/1, Sum3/1
  delta/1 -> Sum5/2, Sum4/2, Sum3/2
  ma/1 -> Product3/1, Product2/1, Product1/1
  Constant2/1 -> Sum5/3
  Sum5/1 -> Trigonometric Function2/1
  Trigonometric Function2/1 -> Product3/2
